simulink model "Sim_Part7"  (R2017b)
settings: Solver=VariableStepAuto  StartTime=0.0  StopTime=100  RelTol=1e-3
settings Model: Creator=Mohammadreza  LastModifiedBy=Mohammadreza

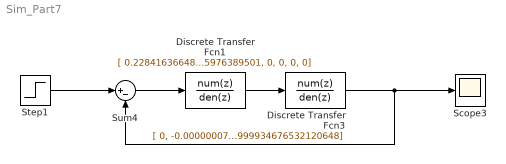
== system Sim_Part7 ==
  Discrete Transfer Fcn1 : DiscreteTransferFcn  Numerator=[ 0.228416366489491706737169351982, 0.178587336139809038648706973618, -1.49566837490891924034031035262, 1.57129347654044382309734828596, -0.482628804260825605698670415222, 0, 0, 0, 0]  Denominator=[ -0.0000000700000000000000047733017083211, -0.000000236991764345735581868667156587, 0.0000000559816025094406969985420363233, 0.00000020794481383892534326438428921, 0.0000000430653479973695397615976389501, 0, 0, 0, 0]  SampleTime=4
  Discrete Transfer Fcn3 : DiscreteTransferFcn  Numerator=[ 0, -0.0000000700000000000000047733017083211, -0.000000252980909999999998403775189684, -0.0000000558142320897000021751117242001]  Denominator=[ 1.0, -2.59612, 2.22162420110000002893002601922, -0.625504201099999934676532120648]  SampleTime=4
  Scope3 : Scope
  Step1 : Step  Time=0  SampleTime=0
  Sum4 : Sum  Inputs=|+-
  wires:
  Step1/1 -> Sum4/1
  Discrete Transfer Fcn3/1 -> Scope3/1, Sum4/2
  Sum4/1 -> Discrete Transfer Fcn1/1
  Discrete Transfer Fcn1/1 -> Discrete Transfer Fcn3/1
